simulink model "demostration1_org"  (Simulink 10.0)
settings: Solver=ode4  StartTime=0.0  StopTime=45.77  FixedStep=0.01  RelTol=1e-3
settings Model: Creator=wangze  LastModifiedBy=annonymous
settings DataIOCC: LimitDataPoints=on
settings OptimizationCC: BlockReduction=off  BooleanDataType=off
settings DebuggingCC: SaveWithParameterizedLinksMsg=none  SignalResolutionControl=TryResolveAllWithWarning  AllowSymbolicDim=off
settings HardwareCC: TargetUnknown=on
settings GRTTargetCC: GeneratePreprocessorConditionals=Disable all  CombineOutputUpdateFcns=on  GRTInterface=off
settings ConfigComp: CovExternalEMLEnable=off  CovSFcnEnable=off

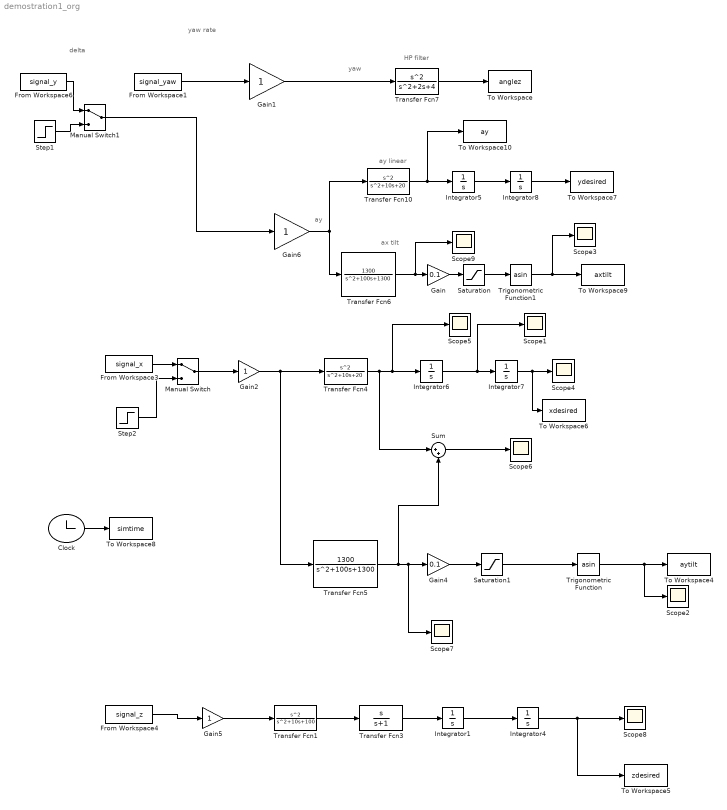
== system demostration1_org ==
  note: ax tilt
  note: ay linear
  note: ay
  note: HP filter
  note: yaw
  note: yaw rate
  note: delta
  Clock : Clock
  From Workspace1 : FromWorkspace  VariableName=signal_yaw  SampleTime=0.01
  From Workspace3 : FromWorkspace  VariableName=signal_x  SampleTime=0.01
  From Workspace4 : FromWorkspace  VariableName=signal_z  SampleTime=0.01
  From Workspace6 : FromWorkspace  VariableName=signal_y  SampleTime=0.01
  Gain : Gain  Gain=0.1
  Gain{1..2,5..6} (4 alike) : Gain
  Gain4 : Gain  Gain=0.1
  Integrator{1,4..8} (6 alike) : Integrator
  Manual Switch : ManualSwitch
  Manual Switch1 : ManualSwitch
  Saturation : Saturate  UpperLimit=1  LowerLimit=-1
  Saturation1 : Saturate  UpperLimit=1  LowerLimit=-1
  Scope{1..9} (9 alike) : Scope
  Step1 : Step  Time=0  SampleTime=0
  Step2 : Step  Time=0  SampleTime=0
  Sum : Sum  Inputs=|++
  To Workspace : ToWorkspace  VariableName=anglez  SampleTime=-1
      settings: Decimation=2
  To Workspace10 : ToWorkspace  VariableName=ay  SampleTime=-1
      settings: Decimation=2
  To Workspace4 : ToWorkspace  VariableName=aytilt  SampleTime=-1
      settings: Decimation=2
  To Workspace5 : ToWorkspace  VariableName=zdesired  SampleTime=-1
      settings: Decimation=2  Save2DSignal=2-D array (concatenate along first dimension)
  To Workspace6 : ToWorkspace  VariableName=xdesired  SampleTime=-1
      settings: Decimation=2  Save2DSignal=2-D array (concatenate along first dimension)
  To Workspace7 : ToWorkspace  VariableName=ydesired  SampleTime=-1
      settings: Decimation=2  Save2DSignal=2-D array (concatenate along first dimension)
  To Workspace8 : ToWorkspace  VariableName=simtime  SampleTime=-1
      settings: Decimation=2  Save2DSignal=2-D array (concatenate along first dimension)
  To Workspace9 : ToWorkspace  VariableName=axtilt  SampleTime=-1
      settings: Decimation=2  Save2DSignal=2-D array (concatenate along first dimension)
  Transfer Fcn1 : TransferFcn  Numerator=[1 0 0]  Denominator=[1 10 100]
  Transfer Fcn10 : TransferFcn  Numerator=[1 0 0]  Denominator=[1 10 20]
  Transfer Fcn3 : TransferFcn  Numerator=[1 0]  Denominator=[1 1]
  Transfer Fcn4 : TransferFcn  Numerator=[1 0 0]  Denominator=[1 10 20]
  Transfer Fcn5 : TransferFcn  Numerator=[1300]  Denominator=[1 100 1300]
  Transfer Fcn6 : TransferFcn  Numerator=[1300]  Denominator=[1 100 1300]
  Transfer Fcn7 : TransferFcn  Numerator=[1 0 0]  Denominator=[1 2 4]
  Trigonometric Function : Trigonometry  Operator=asin
  Trigonometric Function1 : Trigonometry  Operator=asin
  wires:
  Integrator6/1 -> Scope1/1, Integrator7/1
  Transfer Fcn4/1 -> Sum/1, Scope5/1, Integrator6/1
  Integrator7/1 -> To Workspace6/1, Scope4/1
  Gain4/1 -> Saturation1/1
  Transfer Fcn5/1 -> Sum/2, Scope7/1, Gain4/1
  Gain2/1 -> Transfer Fcn5/1, Transfer Fcn4/1
  Manual Switch/1 -> Gain2/1
  From Workspace4/1 -> Gain5/1
  Gain5/1 -> Transfer Fcn1/1
  Transfer Fcn1/1 -> Transfer Fcn3/1
  Transfer Fcn3/1 -> Integrator1/1
  Integrator1/1 -> Integrator4/1
  Integrator4/1 -> To Workspace5/1, Scope8/1
  Step2/1 -> Manual Switch/2
  From Workspace3/1 -> Manual Switch/1
  Sum/1 -> Scope6/1
  Trigonometric Function/1 -> Scope2/1, To Workspace4/1
  Clock/1 -> To Workspace8/1
  Gain1/1 -> Transfer Fcn7/1
  Transfer Fcn7/1 -> To Workspace/1
  Manual Switch1/1 -> Gain6/1
  Transfer Fcn10/1 -> To Workspace10/1, Integrator5/1
  Integrator5/1 -> Integrator8/1
  Integrator8/1 -> To Workspace7/1
  Transfer Fcn6/1 -> Scope9/1, Gain/1
  Gain/1 -> Saturation/1
  Trigonometric Function1/1 -> Scope3/1, To Workspace9/1
  Gain6/1 -> Transfer Fcn6/1, Transfer Fcn10/1
  Saturation/1 -> Trigonometric Function1/1
  Saturation1/1 -> Trigonometric Function/1
  From Workspace6/1 -> Manual Switch1/1
  Step1/1 -> Manual Switch1/2
  From Workspace1/1 -> Gain1/1
